simulink model "SFM_qlpv"  (R2024b)
settings: Solver=VariableStepAuto  StartTime=0.0  StopTime=50  FixedStep=0.1  RelTol=1e-3
undefined symbols (not defined in the file): Lg
settings Model: Creator=rayane benyoucef  LastModifiedBy=y_had
settings SolverCC: AlgebraicLoopSolver=TrustRegion
settings DataIOCC: ReturnWorkspaceOutputs=off
settings DebuggingCC: UnconnectedInputMsg=warning  UnconnectedOutputMsg=warning  UnconnectedLineMsg=warning  ArithmeticOperatorsInVariantConditions=warning
settings ModelReferenceCC: EnableRefExpFcnMdlSchedulingChecks=on
settings SFSimCC: SimUseLocalCustomCode=off  CustomCodeUndefinedFunction=UseInterfaceOnly
settings RTWCC: RTWUseLocalCustomCode=off  GPUComputeCapability=3.5

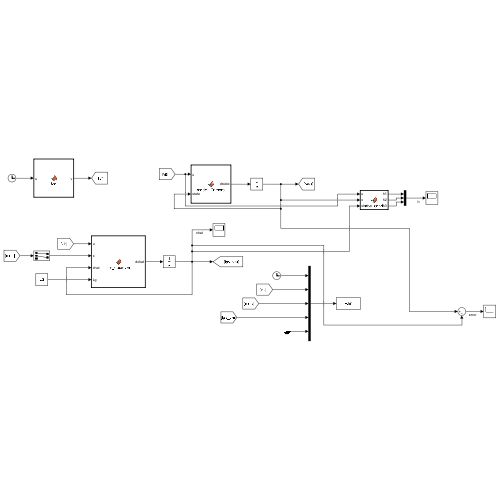
[thumbnail: Simulink's stored preview of the top-level diagram]
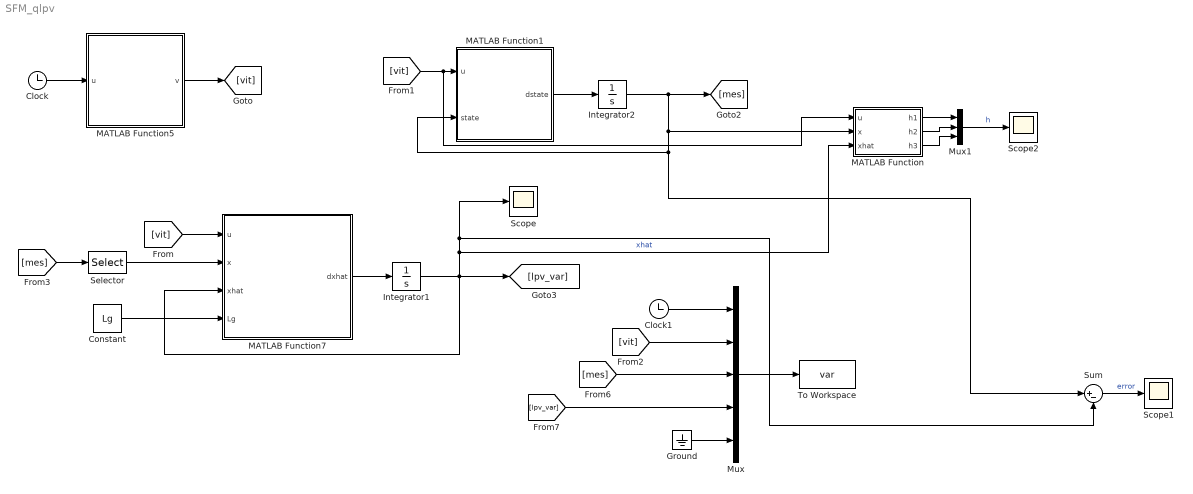
== system SFM_qlpv ==
  Clock : Clock
  Clock1 : Clock
  Constant : Constant  Value=Lg
  Ground : Ground
  Integrator1 : Integrator  InitialCondition=[0.005;.005;0.9]
  Integrator2 : Integrator  InitialCondition=[0.01;0.01;0.9]
  MATLAB Function : MATLAB Function  TreatAsAtomicUnit=on
  MATLAB Function1 : MATLAB Function  TreatAsAtomicUnit=on
  MATLAB Function5 : MATLAB Function  TreatAsAtomicUnit=on
  MATLAB Function7 : MATLAB Function  TreatAsAtomicUnit=on
  Mux : Mux  Inputs=5
  Mux1 : Mux  Inputs=3
  Scope : Scope
  Scope1 : Scope
  Scope2 : Scope
  Selector : Selector  InputPortWidth=3  IndexOptions=Index vector (dialog)  Indices=[1 2]  OutputSizes=1
  Sum : Sum  Inputs=|+-
  To Workspace : ToWorkspace  VariableName=var  SampleTime=-1
  wires:
  Integrator2/1 -> [mes], Sum/1, MATLAB Function1/2(state), MATLAB Function/2(x)
  MATLAB Function1/1(dstate) -> Integrator2/1
  Clock/1 -> MATLAB Function5/1(u)
  Integrator1/1 -> MATLAB Function/3(xhat), Sum/2, Scope/1, [lpv_var], MATLAB Function7/3(xhat)  "xhat"
  MATLAB Function5/1(v) -> [vit]
  [vit] -> MATLAB Function7/1(u)
  [vit] -> MATLAB Function/1(u), MATLAB Function1/1(u)
  [mes] -> Selector/1
  Clock1/1 -> Mux/1
  [vit] -> Mux/2
  [mes] -> Mux/3
  [lpv_var] -> Mux/4
  Mux/1 -> To Workspace/1
  Constant/1 -> MATLAB Function7/4(Lg)
  Selector/1 -> MATLAB Function7/2(x)
  Ground/1 -> Mux/5
  MATLAB Function7/1(dxhat) -> Integrator1/1
  Sum/1 -> Scope1/1  "error"
  MATLAB Function/1(h1) -> Mux1/1
  MATLAB Function/2(h2) -> Mux1/2
  MATLAB Function/3(h3) -> Mux1/3
  Mux1/1 -> Scope2/1  "h"

== matlab function SFM_qlpv/MATLAB Function1 ==
  data: dstate output; u input; state input
function dstate = model_Camera(u,state)

x_img = state(1); y_img = state(2); chi = state(3);

Lint = [-chi 0     x_img*chi  x_img*y_img -(1+x_img^2)  y_img;...
        0    -chi  y_img*chi  1+y_img^2   -x_img*y_img  -x_img;...
        0    0     chi^2      y_img*chi   -x_img*chi    0];


dstate = Lint*u;

end

== matlab function SFM_qlpv/MATLAB Function ==
  data: u input; h1 output; x input; xhat input; h2 output; h3 output
function [h1, h2, h3] = obs_cond(u,x,xhat)

vx = u(1); vy = u(2); vz = u(3);
wx = u(4); wy = u(5); wz = u(6);
x_img = x(1); y_img = x(2); chi_est = xhat(3);

h1 = -vx +x_img*vz;
h2 = -vy + y_img*vz;
h3 = y_img*wx - x_img*wy +chi_est*vz;

== matlab function SFM_qlpv/MATLAB Function5 ==
  data: v output; u input
function v = fcn(u)


vx=-1/5;%0.7*cos(2*pi*u); 
vy=0.1*sin(4*pi*u + pi/2); 
vz=-1/10;%cos(pi*u) ;
wx=0;%0.1*cos(pi/2*u); 
wy=0; 
wz=-0.01-sin(pi*u/2)/5;
v=[vx;vy;vz;wx;wy;wz];

end

== matlab function SFM_qlpv/MATLAB Function7 ==
  data: dxhat output; u input; x input; xhat input; Lg input
function dxhat   = lpv_observer(u,x,xhat,Lg)

vx = u(1); vy = u(2); vz = u(3);
wx = u(4); wy = u(5); wz = u(6);
x_img = x(1); y_img = x(2);
x_est = xhat(1); y_est = xhat(2); chi_est = xhat(3);
omega = [wx;wy;wz];

L1 = Lg(:,1:2); L2 = Lg(:,3:4); L3 = Lg(:,5:6); L4 = Lg(:,7:8);
L5 = Lg(:,9:10); L6 = Lg(:,11:12); L7 = Lg(:,13:14); L8 = Lg(:,15:16);

h1 = -vx +x_img*vz;
h2 = -vy + y_img*vz;
h3 = chi_est*vz + y_img*wx - x_img*wy;

nbr1=-5; max1=5;
nbr2=-5; max2=5;
nbr3=-5; max3=5;


A11=[0 0 max1; 0  0 max2; 0 0 max3];
A21=[0 0 max1; 0  0 max2; 0 0 nbr3];
A31=[0 0 max1; 0  0 nbr2; 0 0 max3];
A41=[0 0 max1; 0  0 nbr2; 0 0 nbr3];
A51=[0 0 nbr1; 0  0 max2; 0 0 max3];
A61=[0 0 nbr1; 0  0 max2; 0 0 nbr3];
A71=[0 0 nbr1; 0  0 nbr2; 0 0 max3];
A81=[0 0 nbr1; 0  0 nbr2; 0 0 nbr3];

F11 = (h1-nbr1)/(max1-nbr1);
F12 = 1 - F11;

F21 = (h2-nbr2)/(max2-nbr2);
F22 = 1 - F21;

F31 = (h3-nbr3)/(max3-nbr3);
F32 = 1 - F31;

N1=F11*F21*F31;
N2=F11*F21*F32;
N3=F11*F22*F31;
N4=F11*F22*F32;
N5=F12*F21*F31;
N6=F12*F21*F32;
N7=F12*F22*F31;
N8=F12*F22*F32;

C=[1,0,0;0,1,0];
err  =  x - C*xhat; 
B=[x_est*y_est -(1+x_est^2) y_est; 1+y_est^2 -x_est*y_est -x_est; 0 0 0 ];
tmp1 = N1*A11+N2*A21+N3*A31+N4*A41+N5*A51+N6*A61+N7*A71+N8*A81;
tmp2 = (N1*L1+N2*L2+N3*L3+N4*L4+N5*L5+N6*L6+N7*L7+N8*L8)*err;
tmp3 = [0;0;vz*chi_est^2];
dxhat = tmp1*xhat + B*omega + tmp2; %+ tmp3;
end
